simulink model "Mo_phong_1"  (R2019a)
settings: Solver=FixedStepAuto  StartTime=0.0  StopTime=25  FixedStep=0.01  RelTol=1e-3
undefined symbols (not defined in the file): magnitude, sigbuilder_block
libraries: mobileRoboticsLib x9, simulink x4
settings Model: Creator=chemi  LastModifiedBy=chemi

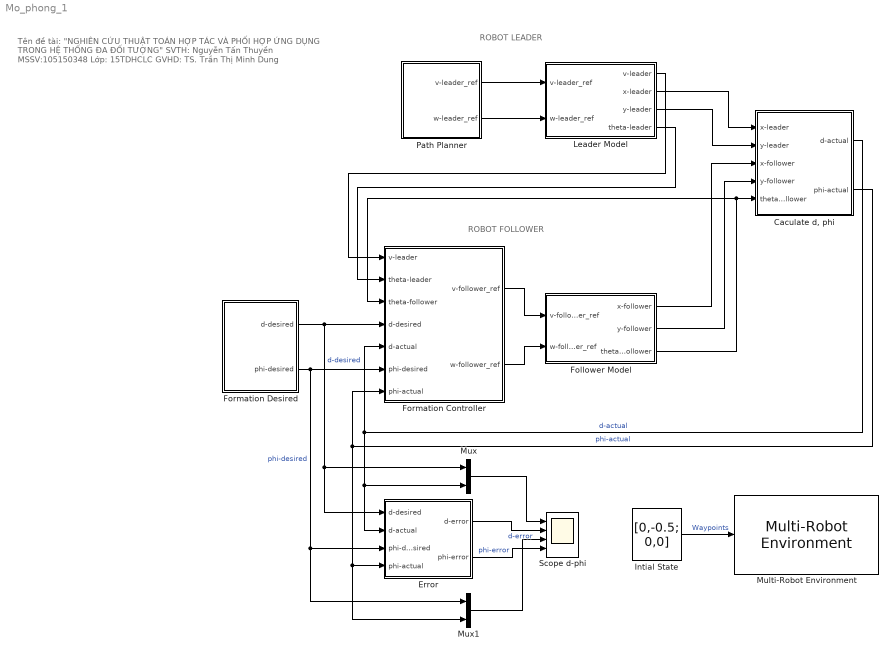
== system Mo_phong_1 ==
  note: ROBOT FOLLOWER
  note: ROBOT LEADER
  note: Tên đề tài: "NGHIÊN CỨU THUẬT TOÁN HỢP TÁC
      | VÀ PHỐI HỢP ỨNG DỤNG TRONG HỆ THỐNG
      | ĐA ĐỐI TƯỢNG"
      |
      | SVTH: Nguyễn Tấn Thuyền MSSV:105150348
      | Lớp: 15TDHCLC
      | GVHD: TS. Trần Thị Minh Dung
  "Caculate d, phi" : Subsystem
  Error : Subsystem
  Follower Model : Subsystem
  Formation Controller : Subsystem
  Formation Desired : Subsystem
  Intial State : Constant  Value=[0,-0.5; 0,0]
  Leader Model : Subsystem
  Multi-Robot Environment : mobileRoboticsLib/Environments/Multi-Robot Environment  numRobots=2  showWaypoints=on  showObjects=off  objectColors=[1 0 0;0 1 0;0 0 1]  objectMarkers='s'  showRobotIds=on  plotSensorLines=off
      settings: SourceProductName=Mobile Robotics Simulation Toolbox
  Mux : Mux  Inputs=2
  Mux1 : Mux  Inputs=2
  Path Planner : Subsystem
  Scope d-phi : Scope  NumInputPorts=4
  wires:
  Path Planner/1(v-leader_ref) -> Leader Model/1(v-leader_ref)
  Intial State/1 -> Multi-Robot Environment/1  "Waypoints"
  Leader Model/2(x-leader) -> "Caculate d, phi"/1(x-leader)
  Follower Model/2(y-follower) -> "Caculate d, phi"/4(y-follower)
  Leader Model/3(y-leader) -> "Caculate d, phi"/2(y-leader)
  Follower Model/1(x-follower) -> "Caculate d, phi"/3(x-follower)
  Follower Model/3(theta-follower) -> "Caculate d, phi"/5(theta-follower), Formation Controller/3(theta-follower)
  "Caculate d, phi"/2(phi-actual) -> Mux1/2, Error/4(phi-actual), Formation Controller/7(phi-actual)  "phi-actual"
  "Caculate d, phi"/1(d-actual) -> Formation Controller/5(d-actual), Mux/2, Error/2(d-actual)  "d-actual"
  Leader Model/1(v-leader) -> Formation Controller/1(v-leader)
  Leader Model/4(theta-leader) -> Formation Controller/2(theta-leader)
  Formation Desired/2(phi-desired) -> Mux1/1, Error/3(phi-desired), Formation Controller/6(phi-desired)  "phi-desired"
  Formation Desired/1(d-desired) -> Mux/1, Error/1(d-desired), Formation Controller/4(d-desired)  "d-desired"
  Formation Controller/1(v-follower_ref) -> Follower Model/1(v-follower_ref)
  Formation Controller/2(w-follower_ref) -> Follower Model/2(w-follower_ref)
  Mux1/1 -> Scope d-phi/3
  Mux/1 -> Scope d-phi/1
  Error/1(d-error) -> Scope d-phi/2  "d-error"
  Error/2(phi-error) -> Scope d-phi/4  "phi-error"
  Path Planner/2(w-leader_ref) -> Leader Model/2(w-leader_ref)

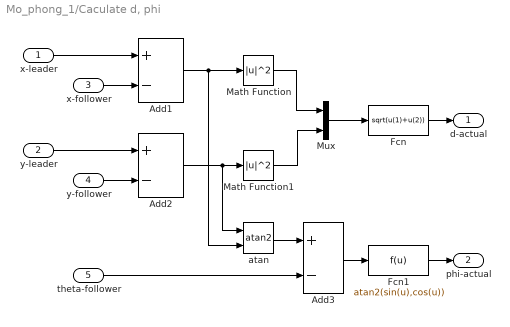
== system Mo_phong_1/Caculate d, phi ==
  x-leader : Inport
  y-leader : Inport  Port=2
  x-follower : Inport  Port=3
  y-follower : Inport  Port=4
  theta-follower : Inport  Port=5
  Add1 : Sum  Inputs=+-
  Add2 : Sum  Inputs=+-
  Add3 : Sum  Inputs=+-
  Fcn : Fcn  Expr=sqrt(u(1)+u(2))
  Fcn1 : Fcn  Expr=atan2(sin(u),cos(u))
  Math Function : Math  Operator=magnitude^2  SaturateOnIntegerOverflow=on
  Math Function1 : Math  Operator=magnitude^2  SaturateOnIntegerOverflow=on
  Mux : Mux  Inputs=2
  atan : Trigonometry  Operator=atan2
  d-actual : Outport
  phi-actual : Outport  Port=2
  wires:
  Math Function1/1 -> Mux/2
  Math Function/1 -> Mux/1
  Mux/1 -> Fcn/1
  Fcn/1 -> d-actual/1
  Add2/1 -> atan/1, Math Function1/1
  Add1/1 -> atan/2, Math Function/1
  x-leader/1 -> Add1/1
  x-follower/1 -> Add1/2
  y-leader/1 -> Add2/1
  y-follower/1 -> Add2/2
  atan/1 -> Add3/1
  theta-follower/1 -> Add3/2
  Add3/1 -> Fcn1/1
  Fcn1/1 -> phi-actual/1

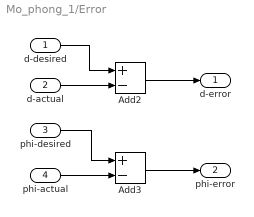
== system Mo_phong_1/Error ==
  d-desired : Inport
  d-actual : Inport  Port=2
  phi-desired : Inport  Port=3
  phi-actual : Inport  Port=4
  Add2 : Sum  Inputs=+-
  Add3 : Sum  Inputs=+-
  d-error : Outport
  phi-error : Outport  Port=2
  wires:
  phi-actual/1 -> Add3/2
  d-actual/1 -> Add2/2
  phi-desired/1 -> Add3/1
  d-desired/1 -> Add2/1
  Add2/1 -> d-error/1
  Add3/1 -> phi-error/1

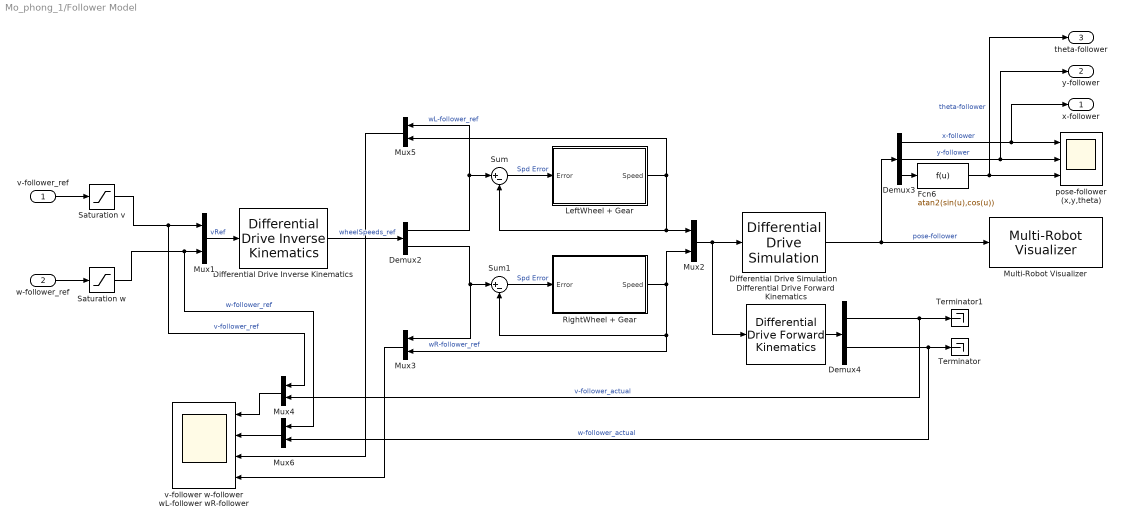
== system Mo_phong_1/Follower Model ==
  v-follower_ref : Inport
  w-follower_ref : Inport  Port=2
  Demux2 : Demux  Outputs=2
  Demux3 : Demux  Outputs=3
  Demux4 : Demux  Outputs=2
  Differential Drive Forward Kinematics : mobileRoboticsLib/Kinematic Models/Differential Drive/Differential Drive Forward Kinematics  wheelRadius=0.0425  wheelBase=0.25
      settings: SourceProductName=Mobile Robotics Simulation Toolbox
  Differential Drive Inverse Kinematics : mobileRoboticsLib/Kinematic Models/Differential Drive/Differential Drive Inverse Kinematics  wheelRadius=0.0425  wheelBase=0.25
      settings: SourceProductName=Mobile Robotics Simulation Library
  Differential Drive Simulation : mobileRoboticsLib/Kinematic Models/Differential Drive/Differential Drive Simulation  wheelRadius=0.0425  wheelBase=0.25  initX=0  initY=-0.5  initAngle=0  Ts=0.01
      settings: SourceProductName=Mobile Robotics Simulation Library
  Fcn6 : Fcn  Expr=atan2(sin(u),cos(u))
  LeftWheel + Gear : Subsystem
  Multi-Robot Visualizer : mobileRoboticsLib/Environments/Multi-Robot Visualizer  idx=2  radius=0.15  robotColor=[0.00 0.45 0.74]  showTraj=on  hasLidar=off  sensorOffset=[0,0]  scanAngles=[-pi/4, 0, pi/4]  hasObjDetector=off  objDetectorOffset=[0,0]  objDetectorAngle=0  objDetectorFOV=pi/3  objDetectorMaxRange=5
      settings: SourceProductName=Mobile Robotics Simulation Toolbox
  Mux{1..6} (6 alike) : Mux  Inputs=2
  RightWheel + Gear : Subsystem
  Saturation v : Saturate  UpperLimit=0.8  LowerLimit=0
  Saturation w : Saturate
  Sum : Sum  Inputs=|+-
  Sum1 : Sum  Inputs=|+-
  Terminator : Terminator
  Terminator1 : Terminator
  pose-follower (x,y,theta) : Scope  NumInputPorts=3
  v-follower w-follower wL-follower wR-follower : Scope  NumInputPorts=4
  x-follower : Outport
  y-follower : Outport  Port=2
  theta-follower : Outport  Port=3
  wires:
  Demux3/2 -> pose-follower (x,y,theta)/2, y-follower/1  "y-follower"
  Differential Drive Simulation/1 -> Multi-Robot Visualizer/1, Demux3/1  "pose-follower"
  Demux3/3 -> Fcn6/1
  Differential Drive Inverse Kinematics/1 -> Demux2/1  "wheelSpeeds_ref"
  v-follower_ref/1 -> Saturation v/1
  Demux3/1 -> pose-follower (x,y,theta)/1, x-follower/1  "x-follower"
  w-follower_ref/1 -> Saturation w/1
  Mux1/1 -> Differential Drive Inverse Kinematics/1  "vRef"
  Demux2/2 -> Mux3/1, Sum1/1  "wR-follower_ref"
  Demux2/1 -> Mux5/1, Sum/1  "wL-follower_ref"
  Sum/1 -> LeftWheel + Gear/1(Error)  "Spd Error"
  LeftWheel + Gear/1(Speed) -> Mux2/1, Sum/2, Mux5/2
  Sum1/1 -> RightWheel + Gear/1(Error)  "Spd Error"
  RightWheel + Gear/1(Speed) -> Mux3/2, Sum1/2, Mux2/2
  Mux2/1 -> Differential Drive Simulation/1, Differential Drive Forward Kinematics/1
  Demux4/2 -> Mux6/2, Terminator/1  "w-follower_actual"
  Differential Drive Forward Kinematics/1 -> Demux4/1
  Demux4/1 -> Terminator1/1, Mux4/2  "v-follower_actual"
  Saturation v/1 -> Mux1/1, Mux4/1  "v-follower_ref"
  Saturation w/1 -> Mux6/1, Mux1/2  "w-follower_ref"
  Fcn6/1 -> pose-follower (x,y,theta)/3, theta-follower/1  "theta-follower"
  Mux4/1 -> v-follower w-follower wL-follower wR-follower/1
  Mux6/1 -> v-follower w-follower wL-follower wR-follower/2
  Mux5/1 -> v-follower w-follower wL-follower wR-follower/3
  Mux3/1 -> v-follower w-follower wL-follower wR-follower/4

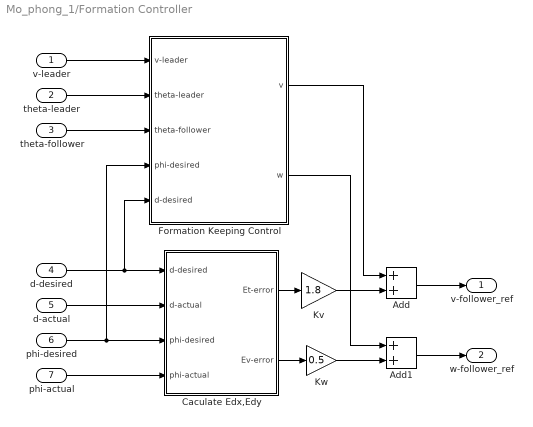
== system Mo_phong_1/Formation Controller ==
  v-leader : Inport
  theta-leader : Inport  Port=2
  theta-follower : Inport  Port=3
  d-desired : Inport  Port=4
  d-actual : Inport  Port=5
  phi-desired : Inport  Port=6
  phi-actual : Inport  Port=7
  Add : Sum
  Add1 : Sum
  Caculate Edx,Edy : Subsystem
  Formation Keeping Control : Subsystem
  Kv : Gain  Gain=1.8
  Kw : Gain  Gain=0.5
  v-follower_ref : Outport
  w-follower_ref : Outport  Port=2
  wires:
  phi-desired/1 -> Formation Keeping Control/4(phi-desired), Caculate Edx,Edy/3(phi-desired)
  theta-follower/1 -> Formation Keeping Control/3(theta-follower)
  Caculate Edx,Edy/1(Et-error) -> Kv/1
  Caculate Edx,Edy/2(Ev-error) -> Kw/1
  theta-leader/1 -> Formation Keeping Control/2(theta-leader)
  d-actual/1 -> Caculate Edx,Edy/2(d-actual)
  v-leader/1 -> Formation Keeping Control/1(v-leader)
  Add/1 -> v-follower_ref/1
  phi-actual/1 -> Caculate Edx,Edy/4(phi-actual)
  Add1/1 -> w-follower_ref/1
  d-desired/1 -> Formation Keeping Control/5(d-desired), Caculate Edx,Edy/1(d-desired)
  Formation Keeping Control/1(v) -> Add/1
  Kv/1 -> Add/2
  Formation Keeping Control/2(w) -> Add1/1
  Kw/1 -> Add1/2

== system Mo_phong_1/Formation Desired ==
  d-ref : Constant  Value=0.5
  phi-ref : Constant  Value=pi/2.05
  d-desired : Outport
  phi-desired : Outport  Port=2
  wires:
  d-ref/1 -> d-desired/1
  phi-ref/1 -> phi-desired/1

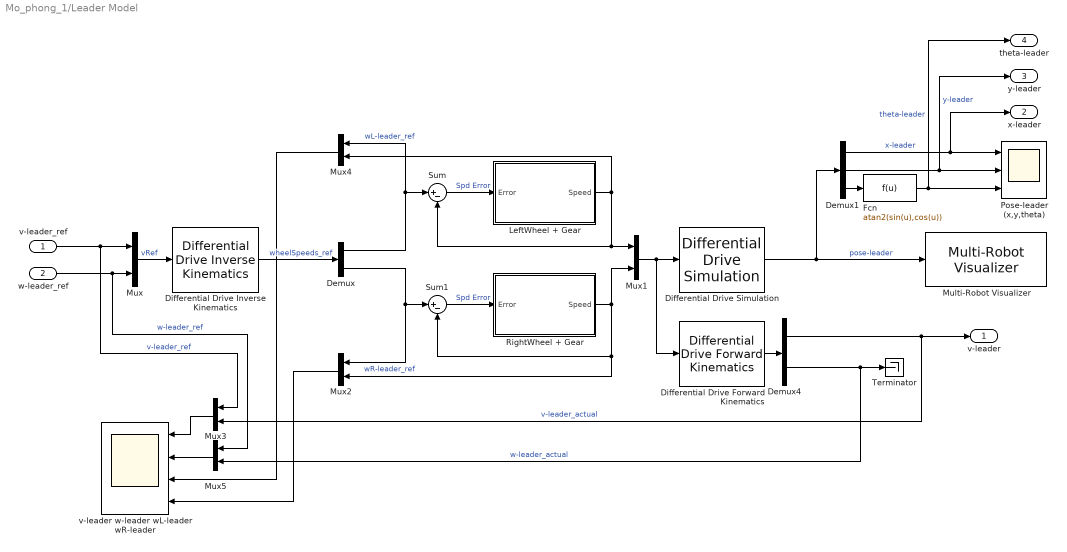
== system Mo_phong_1/Leader Model ==
  v-leader_ref : Inport
  w-leader_ref : Inport  Port=2
  Demux : Demux  Outputs=2
  Demux1 : Demux  Outputs=3
  Demux4 : Demux  Outputs=2
  Differential Drive Forward Kinematics : mobileRoboticsLib/Kinematic Models/Differential Drive/Differential Drive Forward Kinematics  wheelRadius=0.0425  wheelBase=0.25
      settings: SourceProductName=Mobile Robotics Simulation Toolbox
  Differential Drive Inverse Kinematics : mobileRoboticsLib/Kinematic Models/Differential Drive/Differential Drive Inverse Kinematics  wheelRadius=0.0425  wheelBase=0.25
      settings: SourceProductName=Mobile Robotics Simulation Toolbox
  Differential Drive Simulation : mobileRoboticsLib/Kinematic Models/Differential Drive/Differential Drive Simulation  wheelRadius=0.0425  wheelBase=0.25  initX=0  initY=0  initAngle=0  Ts=0.01
      settings: SourceProductName=Mobile Robotics Simulation Toolbox
  Fcn : Fcn  Expr=atan2(sin(u),cos(u))
  LeftWheel + Gear : Subsystem
  Multi-Robot Visualizer : mobileRoboticsLib/Environments/Multi-Robot Visualizer  idx=1  radius=0.15  robotColor=[1.00 0.41 0.16]  showTraj=on  hasLidar=off  sensorOffset=[0,0]  scanAngles=[-pi/4, 0, pi/4]  hasObjDetector=off  objDetectorOffset=[0,0]  objDetectorAngle=0  objDetectorFOV=pi/3  objDetectorMaxRange=5
      settings: SourceProductName=Mobile Robotics Simulation Toolbox
  Mux{,1..5} (6 alike) : Mux  Inputs=2
  Pose-leader (x,y,theta) : Scope  NumInputPorts=3
  RightWheel + Gear : Subsystem
  Sum : Sum  Inputs=|+-
  Sum1 : Sum  Inputs=|+-
  Terminator : Terminator
  v-leader w-leader wL-leader wR-leader : Scope  NumInputPorts=4
  v-leader : Outport
  x-leader : Outport  Port=2
  y-leader : Outport  Port=3
  theta-leader : Outport  Port=4
  wires:
  Differential Drive Inverse Kinematics/1 -> Demux/1  "wheelSpeeds_ref"
  w-leader_ref/1 -> Mux5/1, Mux/2  "w-leader_ref"
  Demux1/3 -> Fcn/1
  Differential Drive Simulation/1 -> Multi-Robot Visualizer/1, Demux1/1  "pose-leader"
  v-leader_ref/1 -> Mux/1, Mux3/1  "v-leader_ref"
  Demux1/2 -> Pose-leader (x,y,theta)/2, y-leader/1  "y-leader"
  Demux1/1 -> Pose-leader (x,y,theta)/1, x-leader/1  "x-leader"
  Demux/1 -> Mux4/1, Sum/1  "wL-leader_ref"
  Demux/2 -> Mux2/1, Sum1/1  "wR-leader_ref"
  Demux4/2 -> Mux5/2, Terminator/1  "w-leader_actual"
  Differential Drive Forward Kinematics/1 -> Demux4/1
  Mux/1 -> Differential Drive Inverse Kinematics/1  "vRef"
  Demux4/1 -> Mux3/2, v-leader/1  "v-leader_actual"
  Sum/1 -> LeftWheel + Gear/1(Error)  "Spd Error"
  LeftWheel + Gear/1(Speed) -> Sum/2, Mux1/1, Mux4/2
  Sum1/1 -> RightWheel + Gear/1(Error)  "Spd Error"
  RightWheel + Gear/1(Speed) -> Mux2/2, Sum1/2, Mux1/2
  Mux1/1 -> Differential Drive Simulation/1, Differential Drive Forward Kinematics/1
  Fcn/1 -> Pose-leader (x,y,theta)/3, theta-leader/1  "theta-leader"
  Mux3/1 -> v-leader w-leader wL-leader wR-leader/1
  Mux4/1 -> v-leader w-leader wL-leader wR-leader/3
  Mux2/1 -> v-leader w-leader wL-leader wR-leader/4
  Mux5/1 -> v-leader w-leader wL-leader wR-leader/2

== system Mo_phong_1/Path Planner ==
  Angular Speed Desired : Subsystem  Tag=STV Subsys  LoadFcn=sigbuilder_block('load');  StartFcn=sigbuilder_block('start');  StopFcn=sigbuilder_block('stop');  ClipboardFcn=sigbuilder_block('clipboard');  mask(Sigbuilder block){tuvar=[0:10]}
      mask help: Simulink:masks:SigbuilderBlock_MD
      mask init:
      | if ~strcmp(get_param(bdroot(gcbh),'SimulationStatus'),'stopped') tuvar = sigbuilder_block('maskInit'); end
      settings: CopyFcn=sigbuilder_block('copy');  DeleteFcn=sigbuilder_block('delete');  ModelCloseFcn=sigbuilder_block('modelClose');  PreSaveFcn=sigbuilder_block('preSave');  PauseFcn=sigbuilder_block('pause');  ContinueFcn=sigbuilder_block('continue');  NameChangeFcn=sigbuilder_block('namechange');  OpenFcn=sigbuilder_block('open',[283.5 152.25 550.5 359.25 ]);  CloseFcn=sigbuilder_block('close');
      mask Display: plot(0, 0, 100, 100,[2, 2, 32, 32, 2], [68, 8, 8, 68, 68],[32, 2], [38, 38], [32, 19, 2],[53, 60, 44], [32, 17, 17, 2],[16, 16, 31, 31]);txt = getActiveGroup(gcbh);text(2, 100, txt,'verticalAlignment', 'top');
  Velocity Desired : Constant  Value=0.4
  Zero-Order Hold : ZeroOrderHold  SampleTime=0.01
  Zero-Order Hold1 : ZeroOrderHold  SampleTime=0.01
  v-leader_ref : Outport
  w-leader_ref : Outport  Port=2
  wires:
  Velocity Desired/1 -> Zero-Order Hold1/1
  Zero-Order Hold/1 -> w-leader_ref/1
  Zero-Order Hold1/1 -> v-leader_ref/1
  Angular Speed Desired/1(Signal 1) -> Zero-Order Hold/1

== system Mo_phong_1/Follower Model/LeftWheel + Gear ==
  Error : Inport
  DC Motor : Subsystem
  Gear : Gain  Gain=1/34
  Speed Controller : Subsystem
  Speed : Outport
  wires:
  Speed Controller/1(Control) -> DC Motor/1(Input)  "Control Input"
  DC Motor/1(Output) -> Gear/1  "Output"
  Gear/1 -> Speed/1
  Error/1 -> Speed Controller/1(Error)

== system Mo_phong_1/Follower Model/RightWheel + Gear ==
  Error : Inport
  DC Motor : Subsystem
  Gear : Gain  Gain=1/34
  Speed Controller : Subsystem
  Speed : Outport
  wires:
  Speed Controller/1(Control) -> DC Motor/1(Input)  "Control Input"
  DC Motor/1(Output) -> Gear/1  "Output"
  Gear/1 -> Speed/1
  Error/1 -> Speed Controller/1(Error)

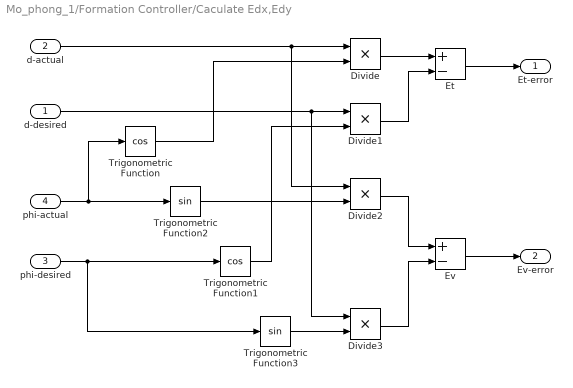
== system Mo_phong_1/Formation Controller/Caculate Edx,Edy ==
  d-desired : Inport
  d-actual : Inport  Port=2
  phi-desired : Inport  Port=3
  phi-actual : Inport  Port=4
  Divide{,1..3} (4 alike) : Product  Inputs=**
  Et : Sum  Inputs=+-
  Ev : Sum  Inputs=+-
  Trigonometric Function : Trigonometry  Operator=cos
  Trigonometric Function1 : Trigonometry  Operator=cos
  Trigonometric Function2 : Trigonometry
  Trigonometric Function3 : Trigonometry
  Et-error : Outport
  Ev-error : Outport  Port=2
  wires:
  d-desired/1 -> Divide1/1, Divide3/1
  d-actual/1 -> Divide/1, Divide2/1
  phi-desired/1 -> Trigonometric Function1/1, Trigonometric Function3/1
  phi-actual/1 -> Trigonometric Function2/1, Trigonometric Function/1
  Trigonometric Function/1 -> Divide/2
  Trigonometric Function1/1 -> Divide1/2
  Divide1/1 -> Et/2
  Divide/1 -> Et/1
  Trigonometric Function2/1 -> Divide2/2
  Trigonometric Function3/1 -> Divide3/2
  Divide3/1 -> Ev/2
  Divide2/1 -> Ev/1
  Et/1 -> Et-error/1
  Ev/1 -> Ev-error/1

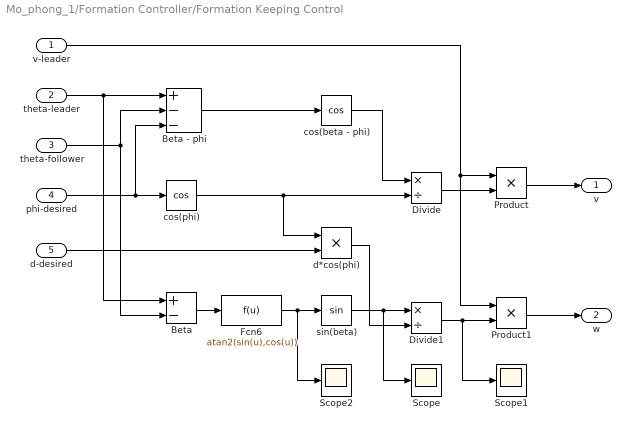
== system Mo_phong_1/Formation Controller/Formation Keeping Control ==
  v-leader : Inport
  theta-leader : Inport  Port=2
  theta-follower : Inport  Port=3
  phi-desired : Inport  Port=4
  d-desired : Inport  Port=5
  Beta : Sum  Inputs=+-
  Beta - phi : Sum  Inputs=+--
  Divide : Product  Inputs=*/
  Divide1 : Product  Inputs=*/
  Fcn6 : Fcn  Expr=atan2(sin(u),cos(u))
  Product : Product
  Product1 : Product
  Scope : Scope
  Scope1 : Scope
  Scope2 : Scope
  cos(beta - phi) : Trigonometry  Operator=cos
  cos(phi) : Trigonometry  Operator=cos
  d*cos(phi) : Product  Inputs=**
  sin(beta) : Trigonometry
  v : Outport
  w : Outport  Port=2
  wires:
  Beta - phi/1 -> cos(beta - phi)/1
  Product/1 -> v/1
  sin(beta)/1 -> Scope/1, Divide1/1
  v-leader/1 -> Product1/1, Product/1
  cos(phi)/1 -> Divide/2, d*cos(phi)/1
  Divide1/1 -> Product1/2, Scope1/1
  theta-leader/1 -> Beta/1, Beta - phi/1
  cos(beta - phi)/1 -> Divide/1
  Divide/1 -> Product/2
  theta-follower/1 -> Beta/2, Beta - phi/2
  Product1/1 -> w/1
  d*cos(phi)/1 -> Divide1/2
  phi-desired/1 -> cos(phi)/1, Beta - phi/3
  d-desired/1 -> d*cos(phi)/2
  Beta/1 -> Fcn6/1
  Fcn6/1 -> Scope2/1, sin(beta)/1

== system Mo_phong_1/Leader Model/LeftWheel + Gear ==
  Error : Inport
  DC Motor : Subsystem
  Gear : Gain  Gain=1/34
  Speed Controller : Subsystem
  Speed : Outport
  wires:
  Speed Controller/1(Control) -> DC Motor/1(Input)  "Control Input"
  DC Motor/1(Output) -> Gear/1  "Output"
  Gear/1 -> Speed/1
  Error/1 -> Speed Controller/1(Error)

== system Mo_phong_1/Leader Model/RightWheel + Gear ==
  Error : Inport
  DC Motor : Subsystem
  Gear : Gain  Gain=1/34
  Speed Controller : Subsystem
  Speed : Outport
  wires:
  Error/1 -> Speed Controller/1(Error)
  Gear/1 -> Speed/1
  DC Motor/1(Output) -> Gear/1  "Output"
  Speed Controller/1(Control) -> DC Motor/1(Input)  "Control Input"

== system Mo_phong_1/Path Planner/Angular Speed Desired ==
  Demux : Demux  Tag=STV Demux  Outputs=1
  FromWs : FromWorkspace  Tag=STV FromWs  VariableName=tuvar  SampleTime=0
      SigBuilderData=|
      | common.afterFinalStr = 'Extrapolate'
      | common.sampleTime = 0
      | dataSet.timeRange = [0 25]
      | dataSet.name = 'Group 1'
      | sbobj.Groups.Name = 'Group 1'
      | sbobj.Groups.Signals.Name = 'Signal 1'
      | sbobj.Groups.Signals.XData = [0 5 5 8 8 15 15 18 18 25]
      | sbobj.Groups.Signals.YData = [0 0 0.25 0.25 0 0 -0.25 -0.25 0 0]
      | sbobj.Groups.TimeRange = [0 25]
  Signal 1 : Outport  Tag=STV Outport
  wires:
  Demux/1 -> Signal 1/1
  FromWs/1 -> Demux/1

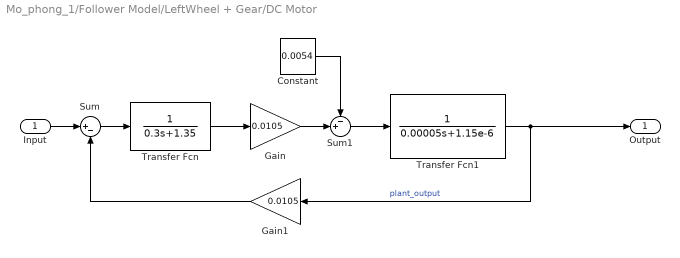
== system Mo_phong_1/Follower Model/LeftWheel + Gear/DC Motor ==
  Input : Inport
  Constant : Constant  Value=0.0054
  Gain : Gain  Gain=0.0105
  Gain1 : Gain  Gain=0.0105
  Sum : Sum  Inputs=|+-
  Sum1 : Sum  Inputs=-+|
  Transfer Fcn : TransferFcn  Denominator=[0.3 1.35]
  Transfer Fcn1 : TransferFcn  Denominator=[0.00005 1.15e-6]
  Output : Outport
  wires:
  Transfer Fcn1/1 -> Gain1/1, Output/1  "plant_output"
  Input/1 -> Sum/1
  Sum/1 -> Transfer Fcn/1
  Transfer Fcn/1 -> Gain/1
  Gain/1 -> Sum1/2
  Sum1/1 -> Transfer Fcn1/1
  Constant/1 -> Sum1/1
  Gain1/1 -> Sum/2

== system Mo_phong_1/Follower Model/LeftWheel + Gear/Speed Controller ==
  Error : Inport
  1-D Lookup Table1 : Lookup_n-D  NumberOfTableDimensions=1  BreakpointsForDimension1=[-255:1:255]  Table=[-11.999994:0.0470588:11.999994]  InternalRulePriority=Speed  RndMeth=Simplest  InputSameDT=on
  PID Controller : simulink/Continuous/PID Controller  Controller=PID  Form=Parallel  TimeDomain=Discrete-time  SampleTime=0.01  IntegratorMethod=Forward Euler  FilterMethod=Forward Euler  ControllerParametersSource=internal  P=48  I=45  D=8.5  UseFilter=off  N=100  TunerSelectOption=Transfer Function Based (PID Tuner App)  InitialConditionSource=internal  InitialConditionForIntegrator=0  InitialConditionForFilter=0  DifferentiatorICPrevScaledInput=0  ExternalReset=none  TrackingMode=off  Kt=1  LimitOutput=on  UpperSaturationLimit=255  LowerSaturationLimit=-255  LinearizeAsGain=on  AntiWindupMode=none  Kb=1  POutMin=[]  POutMax=[]  IOutMin=[]  IOutMax=[]  DOutMin=[]  DOutMax=[]  NOutMin=[]  NOutMax=[]  SumOutMin=[]  SumOutMax=[]  SaturationOutMin=[]  SaturationOutMax=[]  PParamMin=[]  PParamMax=[]  IParamMin=[]  IParamMax=[]  DParamMin=[]  DParamMax=[]  NParamMin=[]  NParamMax=[]  KbParamMin=[]  KbParamMax=[]  KtParamMin=[]  KtParamMax=[]  KbOutMin=[]  KbOutMax=[]  KtOutMin=[]  KtOutMax=[]  IntegratorOutMin=[]  IntegratorOutMax=[]  FilterOutMin=[]  FilterOutMax=[]  SumI1OutMin=[]  SumI1OutMax=[]  SumI2OutMin=[]  SumI2OutMax=[]  SumI3OutMin=[]  SumI3OutMax=[]  SumI4OutMin=[]  SumI4OutMax=[]  SumDOutMin=[]  SumDOutMax=[]  DifferentiatorOutMin=[]  DifferentiatorOutMax=[]  FilterDiffOutCoefMin=[]  FilterDiffOutCoefMax=[]  ReciprocalOutMin=[]  ReciprocalOutMax=[]  SumDenOutMin=[]  SumDenOutMax=[]  SumNumOutMin=[]  SumNumOutMax=[]  DivideOutMin=[]  DivideOutMax=[]  IntegratorContinuousStateAttributes=''  IntegratorStateMustResolveToSignalObject=off  IntegratorRTWStateStorageClass=Auto  FilterContinuousStateAttributes=''  FilterStateMustResolveToSignalObject=off  FilterRTWStateStorageClass=Auto  ParallelPVariant=InternalParameters  IdealPVariant=Disabled  IVariant=InternalParameters  DVariant=InternalParameters  IntegratorVariant=Discrete  SatVariant=Enabled  AWVariant=Passthrough  PCopyVariant=Disabled  TRVariant=Disabled  FdbkBlocksVariant=Forward  IdealPFdbkVariant=Disabled  SatFdbkVariant=Disabled  DerivativeFilterVariant=Differentiator  NVariant=Passthrough  NCopyVariant=Disabled_SignalSpec  FilterICVariant=InternalICsDifferentiator  IntegratorICVariant=InternalICs  ExternalResetVariant=Disabled  TRSumVariant=Passthrough  SumFdbkVariant=Disabled  SumVariant=Sum_PID
  Control : Outport
  wires:
  Error/1 -> PID Controller/1
  PID Controller/1 -> 1-D Lookup Table1/1
  1-D Lookup Table1/1 -> Control/1

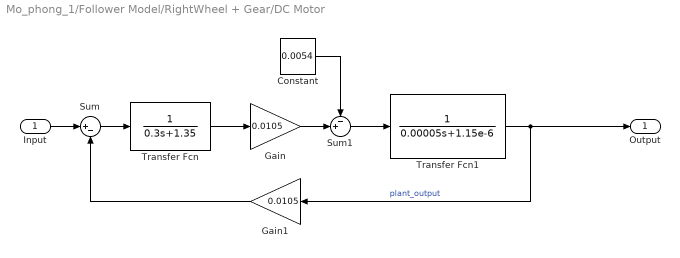
== system Mo_phong_1/Follower Model/RightWheel + Gear/DC Motor ==
  Input : Inport
  Constant : Constant  Value=0.0054
  Gain : Gain  Gain=0.0105
  Gain1 : Gain  Gain=0.0105
  Sum : Sum  Inputs=|+-
  Sum1 : Sum  Inputs=-+|
  Transfer Fcn : TransferFcn  Denominator=[0.3 1.35]
  Transfer Fcn1 : TransferFcn  Denominator=[0.00005 1.15e-6]
  Output : Outport
  wires:
  Transfer Fcn1/1 -> Gain1/1, Output/1  "plant_output"
  Input/1 -> Sum/1
  Sum/1 -> Transfer Fcn/1
  Transfer Fcn/1 -> Gain/1
  Gain/1 -> Sum1/2
  Sum1/1 -> Transfer Fcn1/1
  Constant/1 -> Sum1/1
  Gain1/1 -> Sum/2

== system Mo_phong_1/Follower Model/RightWheel + Gear/Speed Controller ==
  Error : Inport
  1-D Lookup Table1 : Lookup_n-D  NumberOfTableDimensions=1  BreakpointsForDimension1=[-255:1:255]  Table=[-11.999994:0.0470588:11.999994]  InternalRulePriority=Speed  RndMeth=Simplest  InputSameDT=on
  PID Controller : simulink/Continuous/PID Controller  Controller=PID  Form=Parallel  TimeDomain=Discrete-time  SampleTime=0.01  IntegratorMethod=Forward Euler  FilterMethod=Forward Euler  ControllerParametersSource=internal  P=48  I=45  D=8.5  UseFilter=off  N=100  TunerSelectOption=Transfer Function Based (PID Tuner App)  InitialConditionSource=internal  InitialConditionForIntegrator=0  InitialConditionForFilter=0  DifferentiatorICPrevScaledInput=0  ExternalReset=none  TrackingMode=off  Kt=1  LimitOutput=on  UpperSaturationLimit=255  LowerSaturationLimit=-255  LinearizeAsGain=on  AntiWindupMode=none  Kb=1  POutMin=[]  POutMax=[]  IOutMin=[]  IOutMax=[]  DOutMin=[]  DOutMax=[]  NOutMin=[]  NOutMax=[]  SumOutMin=[]  SumOutMax=[]  SaturationOutMin=[]  SaturationOutMax=[]  PParamMin=[]  PParamMax=[]  IParamMin=[]  IParamMax=[]  DParamMin=[]  DParamMax=[]  NParamMin=[]  NParamMax=[]  KbParamMin=[]  KbParamMax=[]  KtParamMin=[]  KtParamMax=[]  KbOutMin=[]  KbOutMax=[]  KtOutMin=[]  KtOutMax=[]  IntegratorOutMin=[]  IntegratorOutMax=[]  FilterOutMin=[]  FilterOutMax=[]  SumI1OutMin=[]  SumI1OutMax=[]  SumI2OutMin=[]  SumI2OutMax=[]  SumI3OutMin=[]  SumI3OutMax=[]  SumI4OutMin=[]  SumI4OutMax=[]  SumDOutMin=[]  SumDOutMax=[]  DifferentiatorOutMin=[]  DifferentiatorOutMax=[]  FilterDiffOutCoefMin=[]  FilterDiffOutCoefMax=[]  ReciprocalOutMin=[]  ReciprocalOutMax=[]  SumDenOutMin=[]  SumDenOutMax=[]  SumNumOutMin=[]  SumNumOutMax=[]  DivideOutMin=[]  DivideOutMax=[]  IntegratorContinuousStateAttributes=''  IntegratorStateMustResolveToSignalObject=off  IntegratorRTWStateStorageClass=Auto  FilterContinuousStateAttributes=''  FilterStateMustResolveToSignalObject=off  FilterRTWStateStorageClass=Auto  ParallelPVariant=InternalParameters  IdealPVariant=Disabled  IVariant=InternalParameters  DVariant=InternalParameters  IntegratorVariant=Discrete  SatVariant=Enabled  AWVariant=Passthrough  PCopyVariant=Disabled  TRVariant=Disabled  FdbkBlocksVariant=Forward  IdealPFdbkVariant=Disabled  SatFdbkVariant=Disabled  DerivativeFilterVariant=Differentiator  NVariant=Passthrough  NCopyVariant=Disabled_SignalSpec  FilterICVariant=InternalICsDifferentiator  IntegratorICVariant=InternalICs  ExternalResetVariant=Disabled  TRSumVariant=Passthrough  SumFdbkVariant=Disabled  SumVariant=Sum_PID
  Control : Outport
  wires:
  Error/1 -> PID Controller/1
  PID Controller/1 -> 1-D Lookup Table1/1
  1-D Lookup Table1/1 -> Control/1

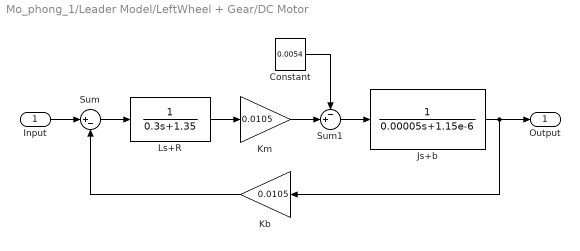
== system Mo_phong_1/Leader Model/LeftWheel + Gear/DC Motor ==
  Input : Inport
  Constant : Constant  Value=0.0054
  Js+b : TransferFcn  Denominator=[0.00005 1.15e-6]
  Kb : Gain  Gain=0.0105
  Km : Gain  Gain=0.0105
  Ls+R : TransferFcn  Denominator=[0.3 1.35]
  Sum : Sum  Inputs=|+-
  Sum1 : Sum  Inputs=-+|
  Output : Outport
  wires:
  Js+b/1 -> Kb/1, Output/1
  Input/1 -> Sum/1
  Sum/1 -> Ls+R/1
  Ls+R/1 -> Km/1
  Km/1 -> Sum1/2
  Sum1/1 -> Js+b/1
  Constant/1 -> Sum1/1
  Kb/1 -> Sum/2

== system Mo_phong_1/Leader Model/LeftWheel + Gear/Speed Controller ==
  Error : Inport
  1-D Lookup Table1 : Lookup_n-D  NumberOfTableDimensions=1  BreakpointsForDimension1=[-255:1:255]  Table=[-11.999994:0.0470588:11.999994]  InternalRulePriority=Speed  RndMeth=Simplest  InputSameDT=on
  PID Controller : simulink/Continuous/PID Controller  Controller=PID  Form=Parallel  TimeDomain=Discrete-time  SampleTime=0.01  IntegratorMethod=Forward Euler  FilterMethod=Forward Euler  ControllerParametersSource=internal  P=28  I=27  D=5  UseFilter=off  N=100  TunerSelectOption=Transfer Function Based (PID Tuner App)  InitialConditionSource=internal  InitialConditionForIntegrator=0  InitialConditionForFilter=0  DifferentiatorICPrevScaledInput=0  ExternalReset=none  TrackingMode=off  Kt=1  LimitOutput=on  UpperSaturationLimit=255  LowerSaturationLimit=-255  LinearizeAsGain=on  AntiWindupMode=none  Kb=1  POutMin=[]  POutMax=[]  IOutMin=[]  IOutMax=[]  DOutMin=[]  DOutMax=[]  NOutMin=[]  NOutMax=[]  SumOutMin=[]  SumOutMax=[]  SaturationOutMin=[]  SaturationOutMax=[]  PParamMin=[]  PParamMax=[]  IParamMin=[]  IParamMax=[]  DParamMin=[]  DParamMax=[]  NParamMin=[]  NParamMax=[]  KbParamMin=[]  KbParamMax=[]  KtParamMin=[]  KtParamMax=[]  KbOutMin=[]  KbOutMax=[]  KtOutMin=[]  KtOutMax=[]  IntegratorOutMin=[]  IntegratorOutMax=[]  FilterOutMin=[]  FilterOutMax=[]  SumI1OutMin=[]  SumI1OutMax=[]  SumI2OutMin=[]  SumI2OutMax=[]  SumI3OutMin=[]  SumI3OutMax=[]  SumI4OutMin=[]  SumI4OutMax=[]  SumDOutMin=[]  SumDOutMax=[]  DifferentiatorOutMin=[]  DifferentiatorOutMax=[]  FilterDiffOutCoefMin=[]  FilterDiffOutCoefMax=[]  ReciprocalOutMin=[]  ReciprocalOutMax=[]  SumDenOutMin=[]  SumDenOutMax=[]  SumNumOutMin=[]  SumNumOutMax=[]  DivideOutMin=[]  DivideOutMax=[]  IntegratorContinuousStateAttributes=''  IntegratorStateMustResolveToSignalObject=off  IntegratorRTWStateStorageClass=Auto  FilterContinuousStateAttributes=''  FilterStateMustResolveToSignalObject=off  FilterRTWStateStorageClass=Auto  ParallelPVariant=InternalParameters  IdealPVariant=Disabled  IVariant=InternalParameters  DVariant=InternalParameters  IntegratorVariant=Discrete  SatVariant=Enabled  AWVariant=Passthrough  PCopyVariant=Disabled  TRVariant=Disabled  FdbkBlocksVariant=Forward  IdealPFdbkVariant=Disabled  SatFdbkVariant=Disabled  DerivativeFilterVariant=Differentiator  NVariant=Passthrough  NCopyVariant=Disabled_SignalSpec  FilterICVariant=InternalICsDifferentiator  IntegratorICVariant=InternalICs  ExternalResetVariant=Disabled  TRSumVariant=Passthrough  SumFdbkVariant=Disabled  SumVariant=Sum_PID
  Control : Outport
  wires:
  Error/1 -> PID Controller/1
  PID Controller/1 -> 1-D Lookup Table1/1
  1-D Lookup Table1/1 -> Control/1

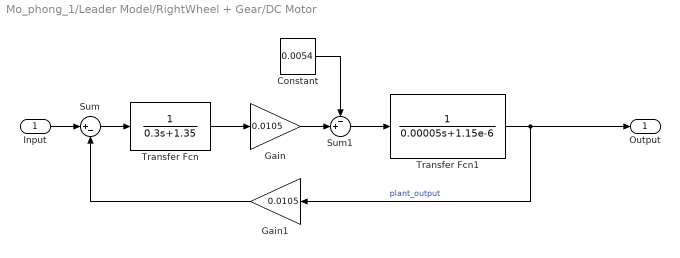
== system Mo_phong_1/Leader Model/RightWheel + Gear/DC Motor ==
  Input : Inport
  Constant : Constant  Value=0.0054
  Gain : Gain  Gain=0.0105
  Gain1 : Gain  Gain=0.0105
  Sum : Sum  Inputs=|+-
  Sum1 : Sum  Inputs=-+|
  Transfer Fcn : TransferFcn  Denominator=[0.3 1.35]
  Transfer Fcn1 : TransferFcn  Denominator=[0.00005 1.15e-6]
  Output : Outport
  wires:
  Gain1/1 -> Sum/2
  Constant/1 -> Sum1/1
  Sum1/1 -> Transfer Fcn1/1
  Gain/1 -> Sum1/2
  Transfer Fcn/1 -> Gain/1
  Sum/1 -> Transfer Fcn/1
  Input/1 -> Sum/1
  Transfer Fcn1/1 -> Output/1, Gain1/1  "plant_output"

== system Mo_phong_1/Leader Model/RightWheel + Gear/Speed Controller ==
  Error : Inport
  1-D Lookup Table1 : Lookup_n-D  NumberOfTableDimensions=1  BreakpointsForDimension1=[-255:1:255]  Table=[-11.999994:0.0470588:11.999994]  InternalRulePriority=Speed  RndMeth=Simplest  InputSameDT=on
  PID Controller : simulink/Continuous/PID Controller  Controller=PID  Form=Parallel  TimeDomain=Discrete-time  SampleTime=0.01  IntegratorMethod=Forward Euler  FilterMethod=Forward Euler  ControllerParametersSource=internal  P=28  I=27  D=5  UseFilter=off  N=100  TunerSelectOption=Transfer Function Based (PID Tuner App)  InitialConditionSource=internal  InitialConditionForIntegrator=0  InitialConditionForFilter=0  DifferentiatorICPrevScaledInput=0  ExternalReset=none  TrackingMode=off  Kt=1  LimitOutput=on  UpperSaturationLimit=255  LowerSaturationLimit=-255  LinearizeAsGain=on  AntiWindupMode=none  Kb=1  POutMin=[]  POutMax=[]  IOutMin=[]  IOutMax=[]  DOutMin=[]  DOutMax=[]  NOutMin=[]  NOutMax=[]  SumOutMin=[]  SumOutMax=[]  SaturationOutMin=[]  SaturationOutMax=[]  PParamMin=[]  PParamMax=[]  IParamMin=[]  IParamMax=[]  DParamMin=[]  DParamMax=[]  NParamMin=[]  NParamMax=[]  KbParamMin=[]  KbParamMax=[]  KtParamMin=[]  KtParamMax=[]  KbOutMin=[]  KbOutMax=[]  KtOutMin=[]  KtOutMax=[]  IntegratorOutMin=[]  IntegratorOutMax=[]  FilterOutMin=[]  FilterOutMax=[]  SumI1OutMin=[]  SumI1OutMax=[]  SumI2OutMin=[]  SumI2OutMax=[]  SumI3OutMin=[]  SumI3OutMax=[]  SumI4OutMin=[]  SumI4OutMax=[]  SumDOutMin=[]  SumDOutMax=[]  DifferentiatorOutMin=[]  DifferentiatorOutMax=[]  FilterDiffOutCoefMin=[]  FilterDiffOutCoefMax=[]  ReciprocalOutMin=[]  ReciprocalOutMax=[]  SumDenOutMin=[]  SumDenOutMax=[]  SumNumOutMin=[]  SumNumOutMax=[]  DivideOutMin=[]  DivideOutMax=[]  IntegratorContinuousStateAttributes=''  IntegratorStateMustResolveToSignalObject=off  IntegratorRTWStateStorageClass=Auto  FilterContinuousStateAttributes=''  FilterStateMustResolveToSignalObject=off  FilterRTWStateStorageClass=Auto  ParallelPVariant=InternalParameters  IdealPVariant=Disabled  IVariant=InternalParameters  DVariant=InternalParameters  IntegratorVariant=Discrete  SatVariant=Enabled  AWVariant=Passthrough  PCopyVariant=Disabled  TRVariant=Disabled  FdbkBlocksVariant=Forward  IdealPFdbkVariant=Disabled  SatFdbkVariant=Disabled  DerivativeFilterVariant=Differentiator  NVariant=Passthrough  NCopyVariant=Disabled_SignalSpec  FilterICVariant=InternalICsDifferentiator  IntegratorICVariant=InternalICs  ExternalResetVariant=Disabled  TRSumVariant=Passthrough  SumFdbkVariant=Disabled  SumVariant=Sum_PID
  Control : Outport
  wires:
  1-D Lookup Table1/1 -> Control/1
  PID Controller/1 -> 1-D Lookup Table1/1
  Error/1 -> PID Controller/1
